simulink library "InputBlocks_library"  (R2018b)
settings: Solver=VariableStepAuto  StartTime=0.0  StopTime=10.0  RelTol=1e-3
undefined symbols (not defined in the file or in its folder): trimPoint
settings Model: Creator=cava_da  LastModifiedBy=cava_da

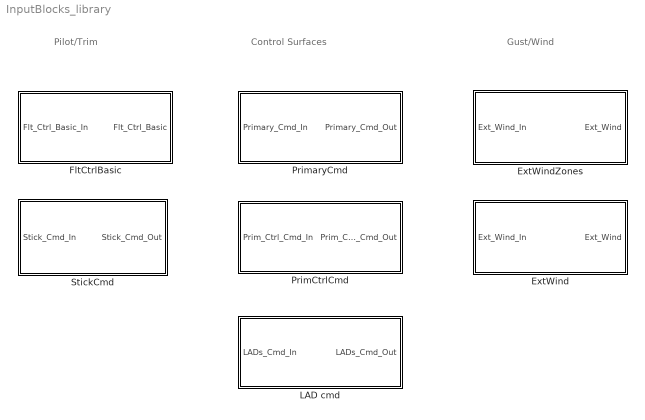
== system InputBlocks_library ==
  note: Gust/Wind
  note: Control Surfaces
  note: Pilot/Trim
  ExtWind : Subsystem
  ExtWindZones : Subsystem
  FltCtrlBasic : Subsystem
  LAD cmd : Subsystem  mask{num_lads=1}
      mask prompts: num_lads "Number of LADs"
      mask DialogControl DescGroupVar Prompt: Load alleviation devices commands
  PrimCtrlCmd : Subsystem
  PrimaryCmd : Subsystem
  StickCmd : Subsystem

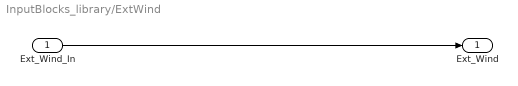
== system InputBlocks_library/ExtWind ==
  Ext_Wind_In : Inport
  Ext_Wind : Outport
  wires:
  Ext_Wind_In/1 -> Ext_Wind/1

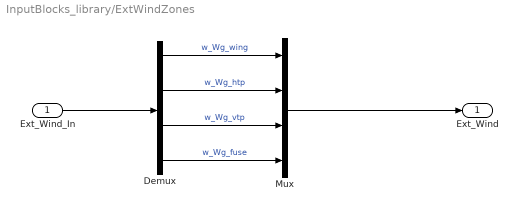
== system InputBlocks_library/ExtWindZones ==
  Ext_Wind_In : Inport
  Demux : Demux
  Mux : Mux
  Ext_Wind : Outport
  wires:
  Ext_Wind_In/1 -> Demux/1
  Demux/1 -> Mux/1  "w_Wg_wing"
  Demux/2 -> Mux/2  "w_Wg_htp"
  Demux/3 -> Mux/3  "w_Wg_vtp"
  Demux/4 -> Mux/4  "w_Wg_fuse"
  Mux/1 -> Ext_Wind/1

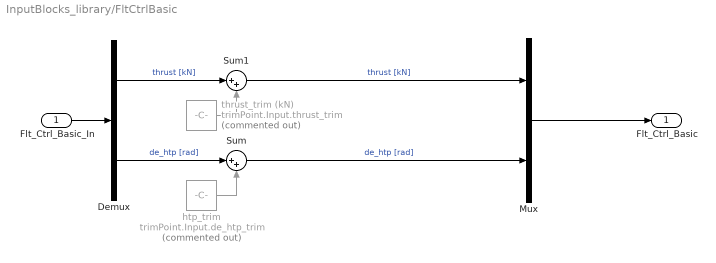
== system InputBlocks_library/FltCtrlBasic ==
  Flt_Ctrl_Basic_In : Inport
  Demux : Demux  Outputs=2
  Mux : Mux  Inputs=2
  Sum : Sum  Inputs=|++
  Sum1 : Sum  Inputs=|++
  htp_trim : Constant  Commented=on  Value=trimPoint.Input.de_htp_trim
  thrust_trim (kN) : Constant  Commented=on  Value=trimPoint.Input.thrust_trim
  Flt_Ctrl_Basic : Outport
  wires:
  Sum/1 -> Mux/2  "de_htp [rad]"
  thrust_trim (kN)/1 -> Sum1/2
  Demux/2 -> Sum/1  "de_htp [rad]"
  htp_trim/1 -> Sum/2
  Demux/1 -> Sum1/1  "thrust [kN]"
  Sum1/1 -> Mux/1  "thrust [kN]"
  Flt_Ctrl_Basic_In/1 -> Demux/1
  Mux/1 -> Flt_Ctrl_Basic/1

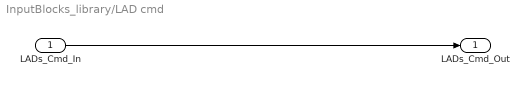
== system InputBlocks_library/LAD cmd ==
  LADs_Cmd_In : Inport  PortDimensions=num_lads
  LADs_Cmd_Out : Outport
  wires:
  LADs_Cmd_In/1 -> LADs_Cmd_Out/1

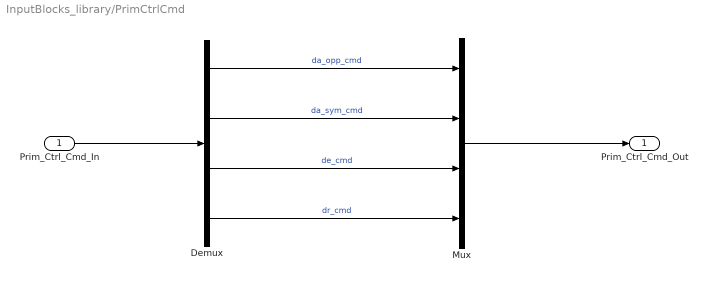
== system InputBlocks_library/PrimCtrlCmd ==
  Prim_Ctrl_Cmd_In : Inport
  Demux : Demux
  Mux : Mux
  Prim_Ctrl_Cmd_Out : Outport
  wires:
  Prim_Ctrl_Cmd_In/1 -> Demux/1
  Mux/1 -> Prim_Ctrl_Cmd_Out/1
  Demux/1 -> Mux/1  "da_opp_cmd"
  Demux/4 -> Mux/4  "dr_cmd"
  Demux/3 -> Mux/3  "de_cmd"
  Demux/2 -> Mux/2  "da_sym_cmd"

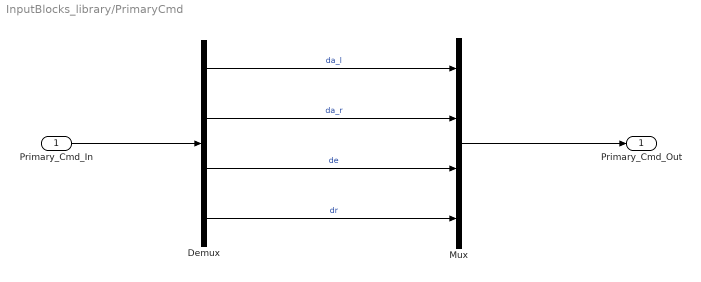
== system InputBlocks_library/PrimaryCmd ==
  Primary_Cmd_In : Inport
  Demux : Demux
  Mux : Mux
  Primary_Cmd_Out : Outport
  wires:
  Primary_Cmd_In/1 -> Demux/1
  Mux/1 -> Primary_Cmd_Out/1
  Demux/1 -> Mux/1  "da_l"
  Demux/4 -> Mux/4  "dr"
  Demux/3 -> Mux/3  "de"
  Demux/2 -> Mux/2  "da_r"

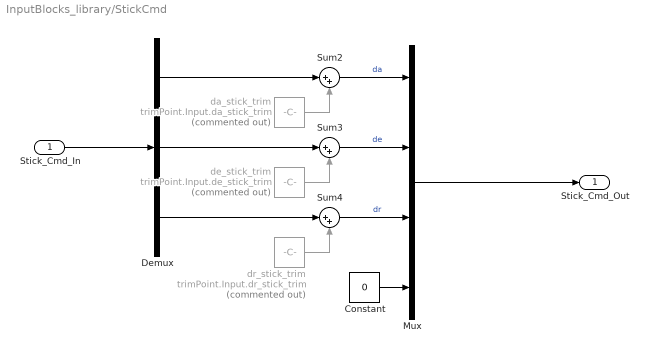
== system InputBlocks_library/StickCmd ==
  Stick_Cmd_In : Inport
  Constant : Constant  Value=0
  Demux : Demux  Outputs=3
  Mux : Mux
  Sum2 : Sum  Inputs=|++
  Sum3 : Sum  Inputs=|++
  Sum4 : Sum  Inputs=|++
  da_stick_trim : Constant  Commented=on  Value=trimPoint.Input.da_stick_trim
  de_stick_trim : Constant  Commented=on  Value=trimPoint.Input.de_stick_trim
  dr_stick_trim : Constant  Commented=on  Value=trimPoint.Input.dr_stick_trim
  Stick_Cmd_Out : Outport
  wires:
  Demux/1 -> Sum2/1
  Constant/1 -> Mux/4
  Sum3/1 -> Mux/2  "de"
  dr_stick_trim/1 -> Sum4/2
  de_stick_trim/1 -> Sum3/2
  Demux/3 -> Sum4/1
  Sum4/1 -> Mux/3  "dr"
  Sum2/1 -> Mux/1  "da"
  da_stick_trim/1 -> Sum2/2
  Demux/2 -> Sum3/1
  Mux/1 -> Stick_Cmd_Out/1
  Stick_Cmd_In/1 -> Demux/1
